simulink model "ZEMAN_Fuzzy_model_A9_NES_2_simulacia"  (R2023b)
settings: Solver=FixedStepAuto  StartTime=0.0  StopTime=20  FixedStep=1e-4  RelTol=1e-4
model workspace (MAT data in the model file):
  A = [0  9; -8  -4]
  B = [13  0; -17  -6]
  C = [1  1; 0  1]
  D = 0
  F1 : sugfis (value not decoded)
  F2 : sugfis (value not decoded)
libraries: fuzblock x2
settings Model: Creator=ivanz  LastModifiedBy=ivanz

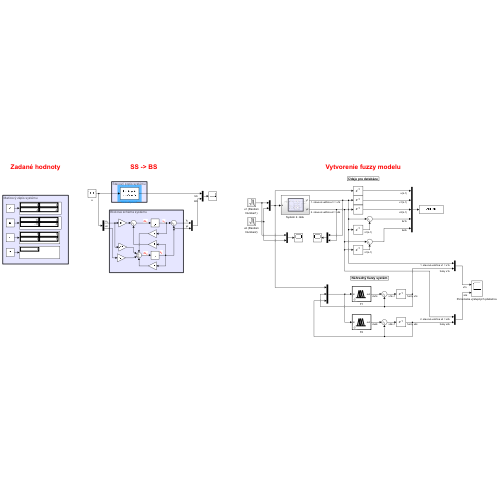
[thumbnail: Simulink's stored preview of the top-level diagram]
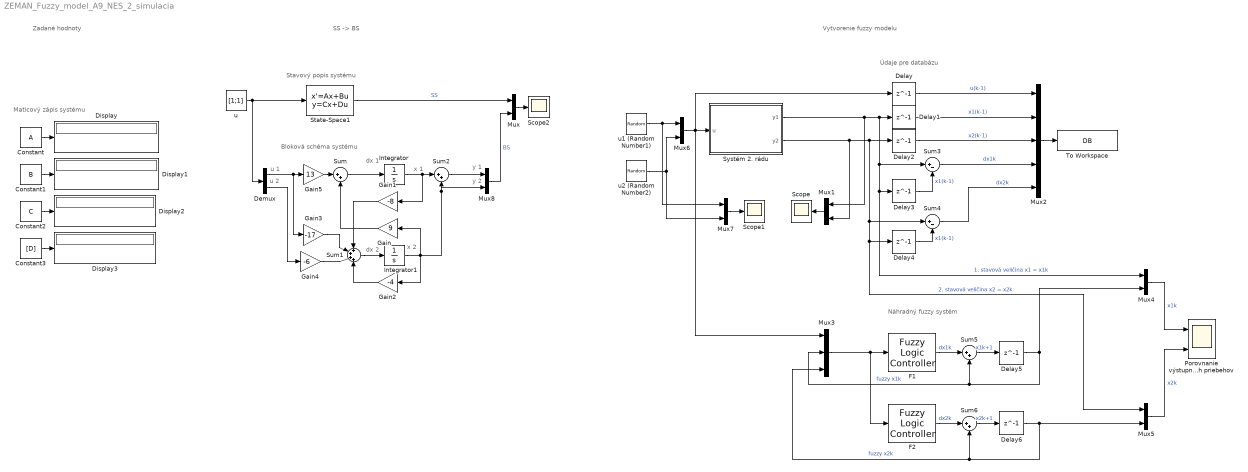
== system ZEMAN_Fuzzy_model_A9_NES_2_simulacia ==
  note: Náhradný fuzzy systém
  note: Údaje pre databázu
  note: Vytvorenie fuzzy modelu
  note: dx 1
  note: Bloková schéma systému
  note: u 1
  note: x 1
  note: Maticový zápis systému
  note: dx 2
  note: Stavový popis systému
  note: y 1
  note: y 2
  note: SS -> BS
  note: x 2
  note: Zadané hodnoty
  note: u 2
  Constant : Constant  Value=A
  Constant1 : Constant  Value=B
  Constant2 : Constant  Value=C
  Constant3 : Constant  Value=[D]
  Delay{,1..6} (7 alike) : Delay  DelayLength=1  InitialCondition=0  SampleTime=0.01
  Demux : Demux  Outputs=2
  Display{,1..3} (4 alike) : Display
  F1 : fuzblock/Fuzzy Logic  Controller  FIS=F1  OutputSampleNumber=101  DataType=double  FuzzifiedInputs=off  RuleFiringStrengths=off  RuleOutputs=off  AggregatedOutputs=off  SimulateUsing=Interpreted execution  OutOfRangeInputValueMessage=warning  NoRuleFiredMessage=warning  EmptyOutputFuzzySetMessage=warning
  F2 : fuzblock/Fuzzy Logic  Controller  FIS=F2  OutputSampleNumber=101  DataType=double  FuzzifiedInputs=off  RuleFiringStrengths=off  RuleOutputs=off  AggregatedOutputs=off  SimulateUsing=Interpreted execution  OutOfRangeInputValueMessage=warning  NoRuleFiredMessage=warning  EmptyOutputFuzzySetMessage=warning
  Gain : Gain  Gain=9
  Gain1 : Gain  Gain=-8
  Gain2 : Gain  Gain=-4
  Gain3 : Gain  Gain=-17
  Gain4 : Gain  Gain=-6
  Gain5 : Gain  Gain=13
  Integrator : Integrator
  Integrator1 : Integrator
  Mux{,1,4..8} (7 alike) : Mux  Inputs=2
  Mux2 : Mux  Inputs=5
  Mux3 : Mux  Inputs=3
  Porovnanie výstupných priebehov : Scope  NumInputPorts=2
  Scope : Scope
  Scope1 : Scope
  Scope2 : Scope
  State-Space1 : StateSpace  A=[A]  B=[B]  C=[C]  D=[0 0; 0 0]  InitialCondition=0
  Sum{,2,5..6} (4 alike) : Sum  Inputs=|++
  Sum1 : Sum  Inputs=++++
  Sum3 : Sum  Inputs=|+-
  Sum4 : Sum  Inputs=|+-
  Systém 2. rádu : Subsystem
  To Workspace : ToWorkspace  VariableName=DB  SampleTime=.01
  u : Constant  Value=[1;1]
  u1 (Random Number1) : RandomNumber  SampleTime=4
  u2 (Random Number2) : RandomNumber  Mean=0.3  Variance=0.8  SampleTime=4
  wires:
  Delay1/1 -> Mux2/2  "x1(k-1)"
  Delay/1 -> Mux2/1  "u(k-1)"
  Delay2/1 -> Mux2/3  "x2(k-1)"
  Mux2/1 -> To Workspace/1
  Mux5/1 -> Porovnanie výstupných priebehov/2  "x2k"
  Mux4/1 -> Porovnanie výstupných priebehov/1  "x1k"
  Sum5/1 -> Delay5/1  "x1k+1"
  F2/1 -> Sum6/1  "dx2k"
  Mux6/1 -> Delay/1, Systém 2. rádu/1(u), Mux3/1
  Delay3/1 -> Sum3/2  "x1(k-1)"
  Delay6/1 -> Mux5/2, Sum6/2, Mux3/3  "fuzzy x2k"
  Delay5/1 -> Mux4/2, Sum5/2, Mux3/2  "fuzzy x1k"
  Systém 2. rádu/1(y1) -> Sum3/1, Mux4/1, Delay3/1, Delay1/1, Mux1/1  "1. stavová veličina x1 = x1k"
  F1/1 -> Sum5/1  "dx1k"
  Systém 2. rádu/2(y2) -> Mux5/1, Delay4/1, Sum4/1, Delay2/1, Mux1/2  "2. stavová veličina x2 = x2k"
  Sum6/1 -> Delay6/1  "x2k+1"
  Sum4/1 -> Mux2/5  "dx2k"
  Sum3/1 -> Mux2/4  "dx1k"
  Mux3/1 -> F1/1, F2/1
  Delay4/1 -> Sum4/2  "x1(k-1)"
  u1 (Random Number1)/1 -> Mux6/1, Mux7/1
  u2 (Random Number2)/1 -> Mux6/2, Mux7/2
  Mux1/1 -> Scope/1
  Mux7/1 -> Scope1/1
  Demux/1 -> Gain3/1, Gain5/1
  Gain3/1 -> Sum1/2
  Gain5/1 -> Sum/1
  Integrator1/1 -> Sum2/2, Mux8/2, Gain/1, Gain2/1
  Mux8/1 -> Mux/2  "BS"
  Integrator/1 -> Gain1/1, Sum2/1
  Sum/1 -> Integrator/1
  Gain/1 -> Sum/2
  Sum1/1 -> Integrator1/1
  Mux/1 -> Scope2/1
  Constant2/1 -> Display2/1
  Constant1/1 -> Display1/1
  State-Space1/1 -> Mux/1  "SS"
  Demux/2 -> Gain4/1
  Constant3/1 -> Display3/1
  Sum2/1 -> Mux8/1
  Constant/1 -> Display/1
  Gain2/1 -> Sum1/4
  u/1 -> Demux/1, State-Space1/1
  Gain4/1 -> Sum1/3
  Gain1/1 -> Sum1/1

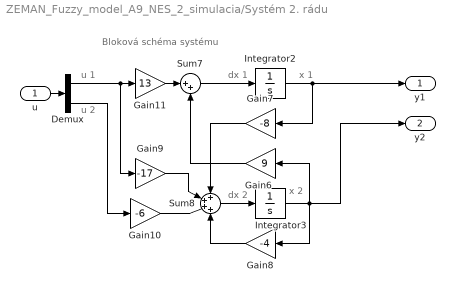
== system ZEMAN_Fuzzy_model_A9_NES_2_simulacia/Systém 2. rádu ==
  note: Bloková schéma systému
  note: dx 2
  note: dx 1
  note: x 1
  note: x 2
  note: u 1
  note: u 2
  u : Inport
  Demux : Demux  Outputs=2
  Gain10 : Gain  Gain=-6
  Gain11 : Gain  Gain=13
  Gain6 : Gain  Gain=9
  Gain7 : Gain  Gain=-8
  Gain8 : Gain  Gain=-4
  Gain9 : Gain  Gain=-17
  Integrator2 : Integrator
  Integrator3 : Integrator
  Sum7 : Sum  Inputs=|++
  Sum8 : Sum  Inputs=++++
  y1 : Outport
  y2 : Outport  Port=2
  wires:
  Sum8/1 -> Integrator3/1
  Gain9/1 -> Sum8/2
  Gain8/1 -> Sum8/4
  Gain6/1 -> Sum7/2
  Integrator3/1 -> y2/1, Gain6/1, Gain8/1
  Gain7/1 -> Sum8/1
  Gain11/1 -> Sum7/1
  Integrator2/1 -> y1/1, Gain7/1
  Gain10/1 -> Sum8/3
  Sum7/1 -> Integrator2/1
  Demux/1 -> Gain9/1, Gain11/1
  Demux/2 -> Gain10/1
  u/1 -> Demux/1
